simulink model "Simscape_Final_08042025"  (R2022a)
settings: Solver=VariableStepAuto  StartTime=0.0  StopTime=180  RelTol=1e-3  AbsTol=1e-3
libraries: fl_lib x30, sh_lib x20, nesl_utility x15, sdl_lib x3
settings Model: Creator=HP  LastModifiedBy=Abhishek
settings SolverCC: AutoScaleAbsTol=off  AlgebraicLoopSolver=TrustRegion  MaxZcPerStep=1
settings DebuggingCC: UnconnectedInputMsg=warning  UnconnectedOutputMsg=warning  UnconnectedLineMsg=warning  SymbolicDimsDataTypeCodeGenerationDiagnostic=none
settings SFSimCC: CustomCodeUndefinedFunction=UseInterfaceOnly
settings RTWCC: DLArmComputeVersion=19.05
settings SimscapeCC: SimscapeLogType=all  SimscapeLogSimulationStatistics=on  SimscapeLogDataHistory=10000

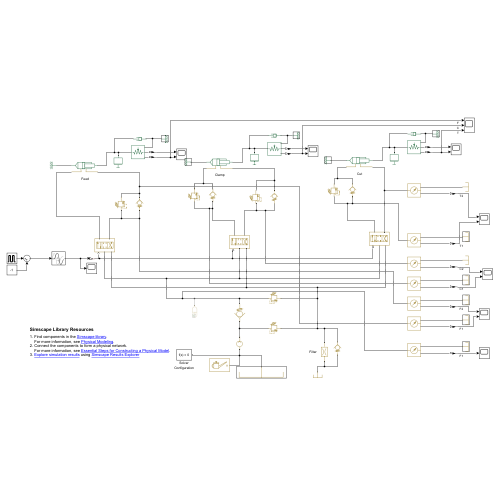
[thumbnail: Simulink's stored preview of the top-level diagram]
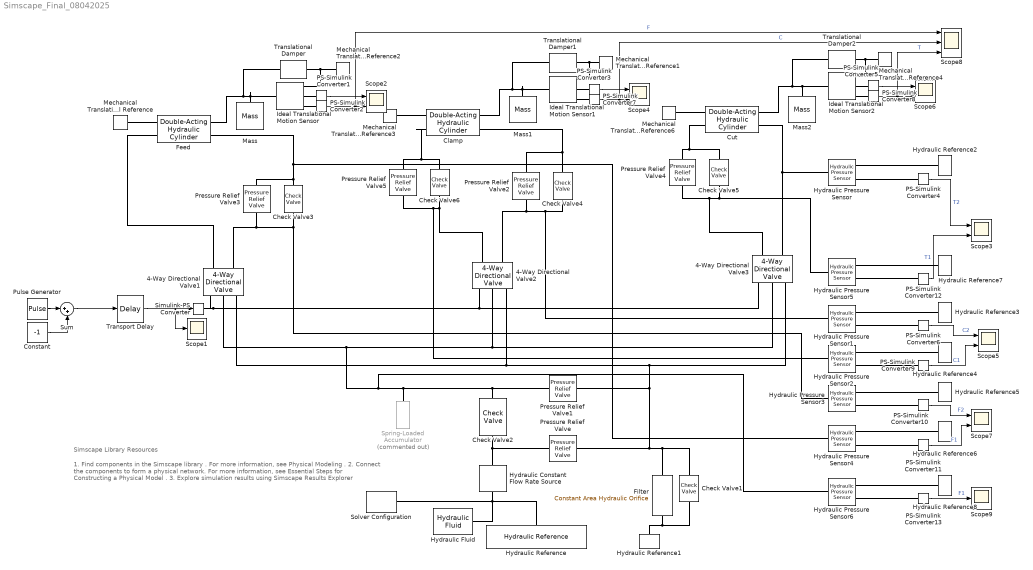
== system Simscape_Final_08042025 ==
  note: 1. Find components in the Simscape library .
      | For more information, see Physical Modeling .
      | 2. Connect the components to form a physical network.
      | For more information, see Essential Steps for Constructing a Physical Model .
      | 3. Explore simulation results using Simscape Results Explorer
  note: Simscape Library Resources
  4-Way Directional Valve1 : sh_lib/Valves/Directional Valves/4-Way Directional Valve  area_spec=sh.valves.directional_valves.enum.area_spec.identical  mdl_type_identical=sh.valves.directional_valves.enum.mdl_type.linear  mdl_type_different=sh.valves.directional_valves.enum.mdl_type.linear  interp_method_identical=sh.valves.directional_valves.enum.interp_method.linear  interp_method_different=sh.valves.directional_valves.enum.interp_method.linear  extrap_method_identical=sh.valves.directional_valves.enum.extrap_method.linear  extrap_method_different=sh.valves.directional_valves.enum.extrap_method.linear  A_leak=1e-12 m^2  C_d=0.7  lam_spec=sh.valves.directional_valves.enum.lam_spec.pressure_ratio  B_lam=0.999  Re_cr=12  opening_max=0.005 m  area_max=0.5e-4 m^2  opening_max_P_A=0.005 m  area_max_P_A=0.5e-4 m^2  opening_max_P_B=0.005 m  area_max_P_B=0.5e-4 m^2  opening_max_A_T=0.005 m  area_max_A_T=0.5e-4 m^2  opening_max_B_T=0.005 m  area_max_B_T=0.5e-4 m^2  opening_area_tab=[-.002, 0, .002, .005, .015] m  area_tab=[1e-09, 2.0352e-07, 4.0736e-05, .00011438, .00034356] m^2  opening_flow_rate_tab=[-.002, 0, .002, .005, .015] m  pressure_tab=[-10000000, -5000000, -2000000, 2000000, 5000000, 10000000] Pa  flow_rate_tab=[-1e-07, -7.0711e-08, -4.4721e-08, 4.4721e-08, 7.0711e-08, 1e-07; -2.0352e-05, -1.4391e-05, -9.1017e-06, 9.1017e-06, 1.4391e-05, 2.0352e-05; -.0040736, -.0028805, -.0018218, .0018218, .0028805, .0040736; -.011438, -.0080879, -.0051152, .0051152, .0080879, .011438; -.034356, -.024293, -.015364, .015364, .024293, .034356] m^3/s  opening_area_tab_P_A=[-.002, 0, .002, .005, .015] m  area_tab_P_A=[1e-09, 2.0352e-07, 4.0736e-05, .00011438, .00034356] m^2  opening_flow_rate_tab_P_A=[-.002, 0, .002, .005, .015] m  pressure_tab_P_A=[-10000000, -5000000, -2000000, 2000000, 5000000, 10000000] Pa  flow_rate_tab_P_A=[-1e-07, -7.0711e-08, -4.4721e-08, 4.4721e-08, 7.0711e-08, 1e-07; -2.0352e-05, -1.4391e-05, -9.1017e-06, 9.1017e-06, 1.4391e-05, 2.0352e-05; -.0040736, -.0028805, -.0018218, .0018218, .0028805, .0040736; -.011438, -.0080879, -.0051152, .0051152, .0080879, .011438; -.034356, -.024293, -.015364, .015364, .024293, .034356] m^3/s  opening_area_tab_P_B=[-.002, 0, .002, .005, .015] m  area_tab_P_B=[1e-09, 2.0352e-07, 4.0736e-05, .00011438, .00034356] m^2  opening_flow_rate_tab_P_B=[-.002, 0, .002, .005, .015] m  pressure_tab_P_B=[-10000000, -5000000, -2000000, 2000000, 5000000, 10000000] Pa  flow_rate_tab_P_B=[-1e-07, -7.0711e-08, -4.4721e-08, 4.4721e-08, 7.0711e-08, 1e-07; -2.0352e-05, -1.4391e-05, -9.1017e-06, 9.1017e-06, 1.4391e-05, 2.0352e-05; -.0040736, -.0028805, -.0018218, .0018218, .0028805, .0040736; -.011438, -.0080879, -.0051152, .0051152, .0080879, .011438; -.034356, -.024293, -.015364, .015364, .024293, .034356] m^3/s  opening_area_tab_A_T=[-.002, 0, .002, .005, .015] m  area_tab_A_T=[1e-09, 2.0352e-07, 4.0736e-05, .00011438, .00034356] m^2  opening_flow_rate_tab_A_T=[-.002, 0, .002, .005, .015] m  pressure_tab_A_T=[-10000000, -5000000, -2000000, 2000000, 5000000, 10000000] Pa  flow_rate_tab_A_T=[-1e-07, -7.0711e-08, -4.4721e-08, 4.4721e-08, 7.0711e-08, 1e-07; -2.0352e-05, -1.4391e-05, -9.1017e-06, 9.1017e-06, 1.4391e-05, 2.0352e-05; -.0040736, -.0028805, -.0018218, .0018218, .0028805, .0040736; -.011438, -.0080879, -.0051152, .0051152, .0080879, .011438; -.034356, -.024293, -.015364, .015364, .024293, .034356] m^3/s  opening_area_tab_B_T=[-.002, 0, .002, .005, .015] m  area_tab_B_T=[1e-09, 2.0352e-07, 4.0736e-05, .00011438, .00034356] m^2  opening_flow_rate_tab_B_T=[-.002, 0, .002, .005, .015] m  pressure_tab_B_T=[-10000000, -5000000, -2000000, 2000000, 5000000, 10000000] Pa  flow_rate_tab_B_T=[-1e-07, -7.0711e-08, -4.4721e-08, 4.4721e-08, 7.0711e-08, 1e-07; -2.0352e-05, -1.4391e-05, -9.1017e-06, 9.1017e-06, 1.4391e-05, 2.0352e-05; -.0040736, -.0028805, -.0018218, .0018218, .0028805, .0040736; -.011438, -.0080879, -.0051152, .0051152, .0080879, .011438; -.034356, -.024293, -.015364, .015364, .024293, .034356] m^3/s  x_0_P_A=0 m  x_0_P_B=0 m  x_0_A_T=0 m  x_0_B_T=0 m
      settings: LogSimulationData=on  InternalSimscapePortConfiguration="{\"Bottom\":[],\"Left\":[{\"id\":\"A\",\"label\":\"A\",\"type\":\"foundation.hydraulic.hydraulic\"},{\"id\":\"B\",\"label\":\"B\",\"type\":\"foundation.hydraulic.hydraulic\"}],\"Right\":[{\"id\":\"S\",\"label\":\"S\",\"type\":\"input\"},{\"id\":\"P\",\"label\":\"P\",\"type\":\"foundation.hydraulic.hydraulic\"},{\"id\":\"T\",\"label\":\"T\",\"type\":\"foundation.hydraulic.hydraulic\"}],\"Top\":[]}"
  4-Way Directional Valve2 : sh_lib/Valves/Directional Valves/4-Way Directional Valve  area_spec=sh.valves.directional_valves.enum.area_spec.identical  mdl_type_identical=sh.valves.directional_valves.enum.mdl_type.linear  mdl_type_different=sh.valves.directional_valves.enum.mdl_type.linear  interp_method_identical=sh.valves.directional_valves.enum.interp_method.linear  interp_method_different=sh.valves.directional_valves.enum.interp_method.linear  extrap_method_identical=sh.valves.directional_valves.enum.extrap_method.linear  extrap_method_different=sh.valves.directional_valves.enum.extrap_method.linear  A_leak=1e-12 m^2  C_d=0.7  lam_spec=sh.valves.directional_valves.enum.lam_spec.pressure_ratio  B_lam=0.999  Re_cr=12  opening_max=0.005 m  area_max=0.5e-4 m^2  opening_max_P_A=0.005 m  area_max_P_A=0.5e-4 m^2  opening_max_P_B=0.005 m  area_max_P_B=0.5e-4 m^2  opening_max_A_T=0.005 m  area_max_A_T=0.5e-4 m^2  opening_max_B_T=0.005 m  area_max_B_T=0.5e-4 m^2  opening_area_tab=[-.002, 0, .002, .005, .015] m  area_tab=[1e-09, 2.0352e-07, 4.0736e-05, .00011438, .00034356] m^2  opening_flow_rate_tab=[-.002, 0, .002, .005, .015] m  pressure_tab=[-10000000, -5000000, -2000000, 2000000, 5000000, 10000000] Pa  flow_rate_tab=[-1e-07, -7.0711e-08, -4.4721e-08, 4.4721e-08, 7.0711e-08, 1e-07; -2.0352e-05, -1.4391e-05, -9.1017e-06, 9.1017e-06, 1.4391e-05, 2.0352e-05; -.0040736, -.0028805, -.0018218, .0018218, .0028805, .0040736; -.011438, -.0080879, -.0051152, .0051152, .0080879, .011438; -.034356, -.024293, -.015364, .015364, .024293, .034356] m^3/s  opening_area_tab_P_A=[-.002, 0, .002, .005, .015] m  area_tab_P_A=[1e-09, 2.0352e-07, 4.0736e-05, .00011438, .00034356] m^2  opening_flow_rate_tab_P_A=[-.002, 0, .002, .005, .015] m  pressure_tab_P_A=[-10000000, -5000000, -2000000, 2000000, 5000000, 10000000] Pa  flow_rate_tab_P_A=[-1e-07, -7.0711e-08, -4.4721e-08, 4.4721e-08, 7.0711e-08, 1e-07; -2.0352e-05, -1.4391e-05, -9.1017e-06, 9.1017e-06, 1.4391e-05, 2.0352e-05; -.0040736, -.0028805, -.0018218, .0018218, .0028805, .0040736; -.011438, -.0080879, -.0051152, .0051152, .0080879, .011438; -.034356, -.024293, -.015364, .015364, .024293, .034356] m^3/s  opening_area_tab_P_B=[-.002, 0, .002, .005, .015] m  area_tab_P_B=[1e-09, 2.0352e-07, 4.0736e-05, .00011438, .00034356] m^2  opening_flow_rate_tab_P_B=[-.002, 0, .002, .005, .015] m  pressure_tab_P_B=[-10000000, -5000000, -2000000, 2000000, 5000000, 10000000] Pa  flow_rate_tab_P_B=[-1e-07, -7.0711e-08, -4.4721e-08, 4.4721e-08, 7.0711e-08, 1e-07; -2.0352e-05, -1.4391e-05, -9.1017e-06, 9.1017e-06, 1.4391e-05, 2.0352e-05; -.0040736, -.0028805, -.0018218, .0018218, .0028805, .0040736; -.011438, -.0080879, -.0051152, .0051152, .0080879, .011438; -.034356, -.024293, -.015364, .015364, .024293, .034356] m^3/s  opening_area_tab_A_T=[-.002, 0, .002, .005, .015] m  area_tab_A_T=[1e-09, 2.0352e-07, 4.0736e-05, .00011438, .00034356] m^2  opening_flow_rate_tab_A_T=[-.002, 0, .002, .005, .015] m  pressure_tab_A_T=[-10000000, -5000000, -2000000, 2000000, 5000000, 10000000] Pa  flow_rate_tab_A_T=[-1e-07, -7.0711e-08, -4.4721e-08, 4.4721e-08, 7.0711e-08, 1e-07; -2.0352e-05, -1.4391e-05, -9.1017e-06, 9.1017e-06, 1.4391e-05, 2.0352e-05; -.0040736, -.0028805, -.0018218, .0018218, .0028805, .0040736; -.011438, -.0080879, -.0051152, .0051152, .0080879, .011438; -.034356, -.024293, -.015364, .015364, .024293, .034356] m^3/s  opening_area_tab_B_T=[-.002, 0, .002, .005, .015] m  area_tab_B_T=[1e-09, 2.0352e-07, 4.0736e-05, .00011438, .00034356] m^2  opening_flow_rate_tab_B_T=[-.002, 0, .002, .005, .015] m  pressure_tab_B_T=[-10000000, -5000000, -2000000, 2000000, 5000000, 10000000] Pa  flow_rate_tab_B_T=[-1e-07, -7.0711e-08, -4.4721e-08, 4.4721e-08, 7.0711e-08, 1e-07; -2.0352e-05, -1.4391e-05, -9.1017e-06, 9.1017e-06, 1.4391e-05, 2.0352e-05; -.0040736, -.0028805, -.0018218, .0018218, .0028805, .0040736; -.011438, -.0080879, -.0051152, .0051152, .0080879, .011438; -.034356, -.024293, -.015364, .015364, .024293, .034356] m^3/s  x_0_P_A=0 m  x_0_P_B=0 m  x_0_A_T=0 m  x_0_B_T=0 m
      settings: LogSimulationData=on  InternalSimscapePortConfiguration="{\"Bottom\":[],\"Left\":[{\"id\":\"A\",\"label\":\"A\",\"type\":\"foundation.hydraulic.hydraulic\"},{\"id\":\"B\",\"label\":\"B\",\"type\":\"foundation.hydraulic.hydraulic\"}],\"Right\":[{\"id\":\"S\",\"label\":\"S\",\"type\":\"input\"},{\"id\":\"P\",\"label\":\"P\",\"type\":\"foundation.hydraulic.hydraulic\"},{\"id\":\"T\",\"label\":\"T\",\"type\":\"foundation.hydraulic.hydraulic\"}],\"Top\":[]}"
  4-Way Directional Valve3 : sh_lib/Valves/Directional Valves/4-Way Directional Valve  area_spec=sh.valves.directional_valves.enum.area_spec.identical  mdl_type_identical=sh.valves.directional_valves.enum.mdl_type.linear  mdl_type_different=sh.valves.directional_valves.enum.mdl_type.linear  interp_method_identical=sh.valves.directional_valves.enum.interp_method.linear  interp_method_different=sh.valves.directional_valves.enum.interp_method.linear  extrap_method_identical=sh.valves.directional_valves.enum.extrap_method.linear  extrap_method_different=sh.valves.directional_valves.enum.extrap_method.linear  A_leak=1e-12 m^2  C_d=0.7  lam_spec=sh.valves.directional_valves.enum.lam_spec.pressure_ratio  B_lam=0.999  Re_cr=12  opening_max=0.005 m  area_max=0.5e-4 m^2  opening_max_P_A=0.005 m  area_max_P_A=0.5e-4 m^2  opening_max_P_B=0.005 m  area_max_P_B=0.5e-4 m^2  opening_max_A_T=0.005 m  area_max_A_T=0.5e-4 m^2  opening_max_B_T=0.005 m  area_max_B_T=0.5e-4 m^2  opening_area_tab=[-.002, 0, .002, .005, .015] m  area_tab=[1e-09, 2.0352e-07, 4.0736e-05, .00011438, .00034356] m^2  opening_flow_rate_tab=[-.002, 0, .002, .005, .015] m  pressure_tab=[-10000000, -5000000, -2000000, 2000000, 5000000, 10000000] Pa  flow_rate_tab=[-1e-07, -7.0711e-08, -4.4721e-08, 4.4721e-08, 7.0711e-08, 1e-07; -2.0352e-05, -1.4391e-05, -9.1017e-06, 9.1017e-06, 1.4391e-05, 2.0352e-05; -.0040736, -.0028805, -.0018218, .0018218, .0028805, .0040736; -.011438, -.0080879, -.0051152, .0051152, .0080879, .011438; -.034356, -.024293, -.015364, .015364, .024293, .034356] m^3/s  opening_area_tab_P_A=[-.002, 0, .002, .005, .015] m  area_tab_P_A=[1e-09, 2.0352e-07, 4.0736e-05, .00011438, .00034356] m^2  opening_flow_rate_tab_P_A=[-.002, 0, .002, .005, .015] m  pressure_tab_P_A=[-10000000, -5000000, -2000000, 2000000, 5000000, 10000000] Pa  flow_rate_tab_P_A=[-1e-07, -7.0711e-08, -4.4721e-08, 4.4721e-08, 7.0711e-08, 1e-07; -2.0352e-05, -1.4391e-05, -9.1017e-06, 9.1017e-06, 1.4391e-05, 2.0352e-05; -.0040736, -.0028805, -.0018218, .0018218, .0028805, .0040736; -.011438, -.0080879, -.0051152, .0051152, .0080879, .011438; -.034356, -.024293, -.015364, .015364, .024293, .034356] m^3/s  opening_area_tab_P_B=[-.002, 0, .002, .005, .015] m  area_tab_P_B=[1e-09, 2.0352e-07, 4.0736e-05, .00011438, .00034356] m^2  opening_flow_rate_tab_P_B=[-.002, 0, .002, .005, .015] m  pressure_tab_P_B=[-10000000, -5000000, -2000000, 2000000, 5000000, 10000000] Pa  flow_rate_tab_P_B=[-1e-07, -7.0711e-08, -4.4721e-08, 4.4721e-08, 7.0711e-08, 1e-07; -2.0352e-05, -1.4391e-05, -9.1017e-06, 9.1017e-06, 1.4391e-05, 2.0352e-05; -.0040736, -.0028805, -.0018218, .0018218, .0028805, .0040736; -.011438, -.0080879, -.0051152, .0051152, .0080879, .011438; -.034356, -.024293, -.015364, .015364, .024293, .034356] m^3/s  opening_area_tab_A_T=[-.002, 0, .002, .005, .015] m  area_tab_A_T=[1e-09, 2.0352e-07, 4.0736e-05, .00011438, .00034356] m^2  opening_flow_rate_tab_A_T=[-.002, 0, .002, .005, .015] m  pressure_tab_A_T=[-10000000, -5000000, -2000000, 2000000, 5000000, 10000000] Pa  flow_rate_tab_A_T=[-1e-07, -7.0711e-08, -4.4721e-08, 4.4721e-08, 7.0711e-08, 1e-07; -2.0352e-05, -1.4391e-05, -9.1017e-06, 9.1017e-06, 1.4391e-05, 2.0352e-05; -.0040736, -.0028805, -.0018218, .0018218, .0028805, .0040736; -.011438, -.0080879, -.0051152, .0051152, .0080879, .011438; -.034356, -.024293, -.015364, .015364, .024293, .034356] m^3/s  opening_area_tab_B_T=[-.002, 0, .002, .005, .015] m  area_tab_B_T=[1e-09, 2.0352e-07, 4.0736e-05, .00011438, .00034356] m^2  opening_flow_rate_tab_B_T=[-.002, 0, .002, .005, .015] m  pressure_tab_B_T=[-10000000, -5000000, -2000000, 2000000, 5000000, 10000000] Pa  flow_rate_tab_B_T=[-1e-07, -7.0711e-08, -4.4721e-08, 4.4721e-08, 7.0711e-08, 1e-07; -2.0352e-05, -1.4391e-05, -9.1017e-06, 9.1017e-06, 1.4391e-05, 2.0352e-05; -.0040736, -.0028805, -.0018218, .0018218, .0028805, .0040736; -.011438, -.0080879, -.0051152, .0051152, .0080879, .011438; -.034356, -.024293, -.015364, .015364, .024293, .034356] m^3/s  x_0_P_A=0 m  x_0_P_B=0 m  x_0_A_T=0 m  x_0_B_T=0 m
      settings: LogSimulationData=on  InternalSimscapePortConfiguration="{\"Bottom\":[],\"Left\":[{\"id\":\"A\",\"label\":\"A\",\"type\":\"foundation.hydraulic.hydraulic\"},{\"id\":\"B\",\"label\":\"B\",\"type\":\"foundation.hydraulic.hydraulic\"}],\"Right\":[{\"id\":\"S\",\"label\":\"S\",\"type\":\"input\"},{\"id\":\"P\",\"label\":\"P\",\"type\":\"foundation.hydraulic.hydraulic\"},{\"id\":\"T\",\"label\":\"T\",\"type\":\"foundation.hydraulic.hydraulic\"}],\"Top\":[]}"
  Check Valve{1..6} (6 alike) : sh_lib/Valves/Directional Valves/Check Valve  area_max=1e-4 m^2  pres_crack=0.3e5 Pa  pres_max=1.2e5 Pa  C_d=0.7  A_leak=1e-12 m^2  lam_spec=1  B_lam=0.999  Re_cr=12  dynamic=0  tau=0.1 s  area_init=1e-12 m^2
      settings: InternalSimscapePortConfiguration="{\"Bottom\":[],\"Left\":[{\"id\":\"A\",\"label\":\"A\",\"type\":\"foundation.hydraulic.hydraulic\"}],\"Right\":[{\"id\":\"B\",\"label\":\"B\",\"type\":\"foundation.hydraulic.hydraulic\"}],\"Top\":[]}"
  Clamp : sh_lib/Hydraulic Cylinders/Double-Acting Hydraulic Cylinder  area_A=1256.6 mm^2  area_B=876.9 mm^2  stroke=150 mm  dead_vol_A=1e-4 m^3  dead_vol_B=1e-4 m^3  k_sh=1.4  or=sh.cylinders.enum.MechOrientationTranslational.Positive  stiff=1e6 N/m  D=150 N*s/m  hardstop_model=1  transition=0.1 mm  displacement_spec=foundation.enum.DisplacementSpec.Calculate  init_pos=0 m  init_pressure_A=0 Pa  init_pressure_B=0 Pa
      settings: InternalSimscapePortConfiguration="{\"Bottom\":[],\"Left\":[{\"id\":\"C\",\"label\":\"C\",\"type\":\"foundation.mechanical.translational.translational\"},{\"id\":\"A\",\"label\":\"A\",\"type\":\"foundation.hydraulic.hydraulic\"}],\"Right\":[{\"id\":\"R\",\"label\":\"R\",\"type\":\"foundation.mechanical.translational.translational\"},{\"id\":\"B\",\"label\":\"B\",\"type\":\"foundation.hydraulic.hydraulic\"}],\"Top\":[]}"
  Constant : Constant  Value=-1
  Cut : sh_lib/Hydraulic Cylinders/Double-Acting Hydraulic Cylinder  area_A=1256.6 mm^2  area_B=876.9 mm^2  stroke=250 mm  dead_vol_A=1e-4 m^3  dead_vol_B=1e-4 m^3  k_sh=1.4  or=sh.cylinders.enum.MechOrientationTranslational.Positive  stiff=1e6 N/m  D=150 N*s/m  hardstop_model=1  transition=0.1 mm  displacement_spec=foundation.enum.DisplacementSpec.Calculate  init_pos=0 m  init_pressure_A=0 Pa  init_pressure_B=0 Pa
      settings: InternalSimscapePortConfiguration="{\"Bottom\":[],\"Left\":[{\"id\":\"C\",\"label\":\"C\",\"type\":\"foundation.mechanical.translational.translational\"},{\"id\":\"A\",\"label\":\"A\",\"type\":\"foundation.hydraulic.hydraulic\"}],\"Right\":[{\"id\":\"R\",\"label\":\"R\",\"type\":\"foundation.mechanical.translational.translational\"},{\"id\":\"B\",\"label\":\"B\",\"type\":\"foundation.hydraulic.hydraulic\"}],\"Top\":[]}"
  Feed : sh_lib/Hydraulic Cylinders/Double-Acting Hydraulic Cylinder  area_A=1256.6 mm^2  area_B=876.9 mm^2  stroke=200 mm  dead_vol_A=1e-4 m^3  dead_vol_B=1e-4 m^3  k_sh=1.4  or=sh.cylinders.enum.MechOrientationTranslational.Positive  stiff=1e6 N/m  D=150 N*s/m  hardstop_model=1  transition=0.1 mm  displacement_spec=foundation.enum.DisplacementSpec.Calculate  init_pos=0 m  init_pressure_A=0 Pa  init_pressure_B=0 Pa
      settings: InternalSimscapePortConfiguration="{\"Bottom\":[],\"Left\":[{\"id\":\"C\",\"label\":\"C\",\"type\":\"foundation.mechanical.translational.translational\"},{\"id\":\"A\",\"label\":\"A\",\"type\":\"foundation.hydraulic.hydraulic\"}],\"Right\":[{\"id\":\"R\",\"label\":\"R\",\"type\":\"foundation.mechanical.translational.translational\"},{\"id\":\"B\",\"label\":\"B\",\"type\":\"foundation.hydraulic.hydraulic\"}],\"Top\":[]}"
  "Filter " : fl_lib/Hydraulic/Hydraulic Elements/Constant Area Hydraulic Orifice  area=1e-4 m^2  C_d=0.7  lam_spec=1  B_lam=0.999  Re_cr=12  q_specify=off  q_priority=None  q=1e-3 m^3/s  q_nominal_specify=off  q_nominal_unit=m^3/s  q_nominal_value=1  p_specify=off  p_priority=None  p=0 Pa  p_nominal_specify=off  p_nominal_unit=Pa  p_nominal_value=1
      settings: InternalSimscapePortConfiguration="{\"Bottom\":[],\"Left\":[{\"id\":\"A\",\"label\":\"A\",\"type\":\"foundation.hydraulic.hydraulic\"}],\"Right\":[{\"id\":\"B\",\"label\":\"B\",\"type\":\"foundation.hydraulic.hydraulic\"}],\"Top\":[]}"
  Hydraulic Constant Flow Rate Source : fl_lib/Hydraulic/Hydraulic Sources/Hydraulic Constant Flow Rate Source  commanded_flow_rate=1.666*0.1*3 gpm
      settings: InternalSimscapePortConfiguration="{\"Bottom\":[],\"Left\":[{\"id\":\"P\",\"label\":\"P\",\"type\":\"foundation.hydraulic.hydraulic\"}],\"Right\":[{\"id\":\"T\",\"label\":\"T\",\"type\":\"foundation.hydraulic.hydraulic\"}],\"Top\":[]}"
  Hydraulic Fluid : sh_lib/Hydraulic Utilities/Hydraulic Fluid  SelFluid=1  SysTemp=60  TrapAir=0.005  ViscDerFactor=1  range_error=2
  Hydraulic Pressure Sensor{,1..6} (7 alike) : fl_lib/Hydraulic/Hydraulic Sensors/Hydraulic Pressure Sensor
  Hydraulic Reference{,1..8} (9 alike) : fl_lib/Hydraulic/Hydraulic Elements/Hydraulic Reference
  Ideal Translational Motion Sensor : fl_lib/Mechanical/Mechanical Sensors/Ideal Translational Motion Sensor  reference=foundation.enum.MeasurementReference.difference  acceleration_port=false  velocity_port=true  position_port=true  offset=0 m
  Ideal Translational Motion Sensor1 : fl_lib/Mechanical/Mechanical Sensors/Ideal Translational Motion Sensor  reference=foundation.enum.MeasurementReference.difference  acceleration_port=false  velocity_port=true  position_port=true  offset=0 m
  Ideal Translational Motion Sensor2 : fl_lib/Mechanical/Mechanical Sensors/Ideal Translational Motion Sensor  reference=foundation.enum.MeasurementReference.difference  acceleration_port=false  velocity_port=true  position_port=true  offset=0 m
  Mass : fl_lib/Mechanical/Translational Elements/Mass  mass=10 kg  num_ports=foundation.enum.numPorts2.one  v_specify=off  v_priority=High  v=0 m/s  v_nominal_specify=off  v_nominal_unit=m/s  v_nominal_value=1  f_specify=off  f_priority=None  f=0 N  f_nominal_specify=off  f_nominal_unit=N  f_nominal_value=1
  Mass1 : fl_lib/Mechanical/Translational Elements/Mass  mass=40 kg  num_ports=foundation.enum.numPorts2.one  v_specify=off  v_priority=High  v=0 m/s  v_nominal_specify=off  v_nominal_unit=m/s  v_nominal_value=1  f_specify=off  f_priority=None  f=0 N  f_nominal_specify=off  f_nominal_unit=N  f_nominal_value=1
  Mass2 : fl_lib/Mechanical/Translational Elements/Mass  mass=80 kg  num_ports=foundation.enum.numPorts2.one  v_specify=off  v_priority=High  v=0 m/s  v_nominal_specify=off  v_nominal_unit=m/s  v_nominal_value=1  f_specify=off  f_priority=None  f=0 N  f_nominal_specify=off  f_nominal_unit=N  f_nominal_value=1
  Mechanical Translational Reference{,1..4,6} (6 alike) : fl_lib/Mechanical/Translational Elements/Mechanical Translational Reference
  PS-Simulink Converter{1..13} (13 alike) : nesl_utility/PS-Simulink Converter  PhysicalDomain=network_engine_domain  SubClassName=ps_output  LeftPortType=input  RightPortType=output  PseudoPeriodic=off  Frequencies=[]  VectorFormat=inherit  Unit=inherit  AffineConversion=off
  Pressure Relief Valve : sh_lib/Valves/Pressure Control Valves/Pressure Relief Valve  valve_area_spec=1  p_diff_TLU=[30.15e5 : 15e3 : 31.35e5] Pa  area_TLU=[1 : 1 : 9] .* 1e-5 m^2  area_max=1e-4 m^2  pres_set=1000 kPa  reg_range=1000*0.2 kPa  C_d=0.7  A_leak=1e-12 m^2  lam_spec=1  B_lam=0.999  Re_cr=12  dynamic=0  tau=0.1 s  area_init=1e-12 m^2
      settings: InternalSimscapePortConfiguration="{\"Bottom\":[],\"Left\":[{\"id\":\"A\",\"label\":\"A\",\"type\":\"foundation.hydraulic.hydraulic\"}],\"Right\":[{\"id\":\"B\",\"label\":\"B\",\"type\":\"foundation.hydraulic.hydraulic\"}],\"Top\":[]}"
  Pressure Relief Valve1 : sh_lib/Valves/Pressure Control Valves/Pressure Relief Valve  valve_area_spec=1  p_diff_TLU=[30.15e5 : 15e3 : 31.35e5] Pa  area_TLU=[1 : 1 : 9] .* 1e-5 m^2  area_max=1e-4 m^2  pres_set=900 kPa  reg_range=900*0.2 kPa  C_d=0.7  A_leak=1e-12 m^2  lam_spec=1  B_lam=0.999  Re_cr=12  dynamic=0  tau=0.1 s  area_init=1e-12 m^2
      settings: InternalSimscapePortConfiguration="{\"Bottom\":[],\"Left\":[{\"id\":\"A\",\"label\":\"A\",\"type\":\"foundation.hydraulic.hydraulic\"}],\"Right\":[{\"id\":\"B\",\"label\":\"B\",\"type\":\"foundation.hydraulic.hydraulic\"}],\"Top\":[]}"
  Pressure Relief Valve2 : sh_lib/Valves/Pressure Control Valves/Pressure Relief Valve  valve_area_spec=1  p_diff_TLU=[30.15e5 : 15e3 : 31.35e5] Pa  area_TLU=[1 : 1 : 9] .* 1e-5 m^2  area_max=1e-4 m^2  pres_set=456 kPa  reg_range=456*0.2 kPa  C_d=0.7  A_leak=1e-12 m^2  lam_spec=1  B_lam=0.999  Re_cr=12  dynamic=0  tau=0.1 s  area_init=1e-12 m^2
      settings: InternalSimscapePortConfiguration="{\"Bottom\":[],\"Left\":[{\"id\":\"A\",\"label\":\"A\",\"type\":\"foundation.hydraulic.hydraulic\"}],\"Right\":[{\"id\":\"B\",\"label\":\"B\",\"type\":\"foundation.hydraulic.hydraulic\"}],\"Top\":[]}"
  Pressure Relief Valve3 : sh_lib/Valves/Pressure Control Valves/Pressure Relief Valve  valve_area_spec=1  p_diff_TLU=[30.15e5 : 15e3 : 31.35e5] Pa  area_TLU=[1 : 1 : 9] .* 1e-5 m^2  area_max=1e-4 m^2  pres_set=750 kPa  reg_range=750*0.2 kPa  C_d=0.7  A_leak=1e-12 m^2  lam_spec=1  B_lam=0.999  Re_cr=12  dynamic=0  tau=0.1 s  area_init=1e-12 m^2
      settings: InternalSimscapePortConfiguration="{\"Bottom\":[],\"Left\":[{\"id\":\"A\",\"label\":\"A\",\"type\":\"foundation.hydraulic.hydraulic\"}],\"Right\":[{\"id\":\"B\",\"label\":\"B\",\"type\":\"foundation.hydraulic.hydraulic\"}],\"Top\":[]}"
  Pressure Relief Valve4 : sh_lib/Valves/Pressure Control Valves/Pressure Relief Valve  valve_area_spec=1  p_diff_TLU=[30.15e5 : 15e3 : 31.35e5] Pa  area_TLU=[1 : 1 : 9] .* 1e-5 m^2  area_max=1e-4 m^2  pres_set=637 kPa  reg_range=127.4 kPa  C_d=0.7  A_leak=1e-12 m^2  lam_spec=1  B_lam=0.999  Re_cr=12  dynamic=0  tau=0.1 s  area_init=1e-12 m^2
      settings: InternalSimscapePortConfiguration="{\"Bottom\":[],\"Left\":[{\"id\":\"A\",\"label\":\"A\",\"type\":\"foundation.hydraulic.hydraulic\"}],\"Right\":[{\"id\":\"B\",\"label\":\"B\",\"type\":\"foundation.hydraulic.hydraulic\"}],\"Top\":[]}"
  Pressure Relief Valve5 : sh_lib/Valves/Pressure Control Valves/Pressure Relief Valve  valve_area_spec=1  p_diff_TLU=[30.15e5 : 15e3 : 31.35e5] Pa  area_TLU=[1 : 1 : 9] .* 1e-5 m^2  area_max=1e-4 m^2  pres_set=318 kPa  reg_range=63 kPa  C_d=0.7  A_leak=1e-12 m^2  lam_spec=1  B_lam=0.999  Re_cr=12  dynamic=0  tau=0.1 s  area_init=1e-12 m^2
      settings: InternalSimscapePortConfiguration="{\"Bottom\":[],\"Left\":[{\"id\":\"A\",\"label\":\"A\",\"type\":\"foundation.hydraulic.hydraulic\"}],\"Right\":[{\"id\":\"B\",\"label\":\"B\",\"type\":\"foundation.hydraulic.hydraulic\"}],\"Top\":[]}"
  Pulse Generator : DiscretePulseGenerator  PulseType=Time based  Amplitude=2  Period=60  PulseWidth=50  PhaseDelay=1
  Scope1 : Scope
  Scope{2..7} (6 alike) : Scope  NumInputPorts=2
  Scope8 : Scope  NumInputPorts=3
  Scope9 : Scope
  Simulink-PS Converter : nesl_utility/Simulink-PS Converter  PhysicalDomain=network_engine_domain  SubClassName=ps_input  LeftPortType=input  RightPortType=output  PseudoPeriodic=off  Frequencies=[]  NoiseDistribution=none  NoiseParameters=[]  Unit=1  AffineConversion=off  FilteringAndDerivatives=provide  SimscapeFilterOrder=1  InputFilterTimeConstant=0.001  UdotUserProvided=0
  Solver Configuration : nesl_utility/Solver Configuration  PhysicalDomain=network_engine_domain  SubClassName=solver  LeftPortType=input  RightPortType=generic  Tones=[]  Harmonics=[]  SimulateNoise=off  Profile=off  UseLocalSampling=off  EnableSwitchedLinearOptims=on  FrequencyDomain=off  UseCCode=off  RelTol=0.001  AbsTol=1e-06  MinStep=1e-09  ToWorkspace=off  RevertToSquareIcSolve=off  NumHomotopyIterations=100  PhasorMode=off  PhasorModeNumHarmonics=1  ConsistencySolver=NEWTON_XTOL_AFTER_FTOL  IndexReductionMethod=DerivativeReplacement  DoDC=off  ResidualTolerance=1e-09  ConsistencyTolSource=GLOBAL  ConsistencyAbsTol=0.001  ConsistencyRelTol=0.001  ConsistencyTolFactor=0.001  UseLocalSolver=off  LocalSolverChoice=NE_BACKWARD_EULER_ADVANCER  ResolveIndetEquations=on  FunctionEvalNumThread=1  LocalSolverSampleTime=0.001  DoFixedCost=off  MaxNonlinIter=3  MaxModeIter=2  ComputeImpulses=off  ImpulseIterations=2  LinearAlgebra=auto  LinearAlgebraNumThread=0  EquationFormulation=NE_TIME_EF  DelaysMemoryBudget=1024  AutomaticFiltering=on  FilteringTimeConstant=0.001  PartitionStorageMethod=AS_NEEDED  PartitionMemoryBudget=1024  PartitionMethod=ROBUST  MultibodyUseLocalSolver=off  MultibodyLocalSolverChoice=ODE1  MultibodyLocalSolverSampleTime=0.001
  Spring-Loaded Accumulator : sh_lib/Accumulators/Spring-Loaded Accumulator  Commented=on  capacity=8 l  pr_preload=400 kPa  pr_max=760 kPa  stiff_coeff=1e12 Pa/m^3  penetr_coeff=1e10 Pa*s/m^6  flow_rate_specify=off  flow_rate_priority=None  flow_rate=5e-3 m^3/s  flow_rate_nominal_specify=off  flow_rate_nominal_unit=m^3/s  flow_rate_nominal_value=1  fluid_volume_specify=on  fluid_volume_priority=High  fluid_volume=5e-3 m^3  fluid_volume_nominal_specify=off  fluid_volume_nominal_unit=m^3  fluid_volume_nominal_value=1  fluid_pressure_specify=off  fluid_pressure_priority=None  fluid_pressure=1.01325e5 Pa  fluid_pressure_nominal_specify=off  fluid_pressure_nominal_unit=Pa  fluid_pressure_nominal_value=1
      settings: InternalSimscapePortConfiguration="{\"Bottom\":[],\"Left\":[],\"Right\":[{\"id\":\"A\",\"label\":\"A\",\"type\":\"foundation.hydraulic.hydraulic\"}],\"Top\":[]}"
  Sum : Sum  Inputs=|++
  Translational Damper : sdl_lib/Couplings & Drives/Springs & Dampers/Translational Damper  D=1000 N*s/m  enable_faults=simscape.enum.onoff.off  b_fault=1e6 N*s/m  temporal_fault=simscape.enum.onoff.off  fault_time=5 s  shock_fault=simscape.enum.onoff.off  acceleration_limit=100 m/s^2  shock_limit=1  report_fault=simscape.enum.assert.action.none  thermal_port=simscape.enum.thermaleffects.omit  thermal_mass=50 kJ/K  temperature_specify=off  temperature_priority=High  temperature=300 K  temperature_nominal_specify=off  temperature_nominal_unit=K  temperature_nominal_value=1
  Translational Damper1 : sdl_lib/Couplings & Drives/Springs & Dampers/Translational Damper  D=1000 N*s/m  enable_faults=simscape.enum.onoff.off  b_fault=1e6 N*s/m  temporal_fault=simscape.enum.onoff.off  fault_time=5 s  shock_fault=simscape.enum.onoff.off  acceleration_limit=100 m/s^2  shock_limit=1  report_fault=simscape.enum.assert.action.none  thermal_port=simscape.enum.thermaleffects.omit  thermal_mass=50 kJ/K  temperature_specify=off  temperature_priority=High  temperature=300 K  temperature_nominal_specify=off  temperature_nominal_unit=K  temperature_nominal_value=1
  Translational Damper2 : sdl_lib/Couplings & Drives/Springs & Dampers/Translational Damper  D=1100 N*s/m  enable_faults=simscape.enum.onoff.off  b_fault=1e6 N*s/m  temporal_fault=simscape.enum.onoff.off  fault_time=5 s  shock_fault=simscape.enum.onoff.off  acceleration_limit=100 m/s^2  shock_limit=1  report_fault=simscape.enum.assert.action.none  thermal_port=simscape.enum.thermaleffects.omit  thermal_mass=50 kJ/K  temperature_specify=off  temperature_priority=High  temperature=300 K  temperature_nominal_specify=off  temperature_nominal_unit=K  temperature_nominal_value=1
  Transport Delay : TransportDelay  DelayTime=60
  wires:
  Constant/1 -> Sum/2
  Sum/1 -> Transport Delay/1
  Pulse Generator/1 -> Sum/1
  PS-Simulink Converter1/1 -> Scope2/1
  PS-Simulink Converter7/1 -> Scope8/2, Scope4/2  "C"
  PS-Simulink Converter3/1 -> Scope4/1
  PS-Simulink Converter8/1 -> Scope8/3, Scope6/2  "T"
  PS-Simulink Converter5/1 -> Scope6/1
  PS-Simulink Converter2/1 -> Scope8/1, Scope2/2  "F"
  PS-Simulink Converter4/1 -> Scope3/1  "T2"
  PS-Simulink Converter6/1 -> Scope5/1  "C2"
  PS-Simulink Converter9/1 -> Scope5/2  "C1"
  PS-Simulink Converter10/1 -> Scope7/1  "F2"
  PS-Simulink Converter11/1 -> Scope7/2  "F1"
  PS-Simulink Converter12/1 -> Scope3/2  "T1"
  PS-Simulink Converter13/1 -> Scope9/1  "F1"
  Transport Delay/1 -> Scope1/1, Simulink-PS Converter/1
  connections:
  Hydraulic Reference/LConn1 -- Solver Configuration/RConn1 -- Hydraulic Fluid/RConn1 -- Hydraulic Constant Flow Rate Source/RConn1
  Hydraulic Constant Flow Rate Source/LConn1 -- Check Valve2/LConn1 -- Pressure Relief Valve/LConn1
  Pressure Relief Valve1/RConn1 -- 4-Way Directional Valve3/RConn3 -- 4-Way Directional Valve2/RConn3 -- 4-Way Directional Valve1/RConn3 -- Pressure Relief Valve/RConn1 -- "Filter "/LConn1 -- Check Valve1/LConn1
  Check Valve1/RConn1 -- Hydraulic Reference1/LConn1 -- "Filter "/RConn1
  Check Valve3/LConn1 -- Feed/RConn2 -- Hydraulic Pressure Sensor4/LConn1 -- Pressure Relief Valve3/RConn1
  Mass/LConn1 -- Translational Damper/LConn1 -- Feed/RConn1 -- Ideal Translational Motion Sensor/LConn1
  Mechanical Translational Reference/LConn1 -- Feed/LConn1
  Simulink-PS Converter/RConn1 -- 4-Way Directional Valve3/RConn1 -- 4-Way Directional Valve2/RConn1 -- 4-Way Directional Valve1/RConn1
  Translational Damper/RConn1 -- Ideal Translational Motion Sensor/RConn1 -- Mechanical Translational Reference2/LConn1
  PS-Simulink Converter2/LConn1 -- Ideal Translational Motion Sensor/RConn3
  PS-Simulink Converter1/LConn1 -- Ideal Translational Motion Sensor/RConn2
  4-Way Directional Valve2/LConn2 -- Hydraulic Pressure Sensor1/LConn1 -- Check Valve4/RConn1 -- Pressure Relief Valve2/LConn1
  Check Valve4/LConn1 -- Pressure Relief Valve2/RConn1 -- Clamp/RConn2
  Mechanical Translational Reference3/LConn1 -- Clamp/LConn1
  Mechanical Translational Reference6/LConn1 -- Cut/LConn1
  Translational Damper1/LConn1 -- Clamp/RConn1 -- Mass1/LConn1 -- Ideal Translational Motion Sensor1/LConn1
  PS-Simulink Converter7/LConn1 -- Ideal Translational Motion Sensor1/RConn3
  PS-Simulink Converter3/LConn1 -- Ideal Translational Motion Sensor1/RConn2
  Translational Damper2/LConn1 -- Cut/RConn1 -- Mass2/LConn1 -- Ideal Translational Motion Sensor2/LConn1
  Ideal Translational Motion Sensor2/RConn3 -- PS-Simulink Converter8/LConn1
  PS-Simulink Converter5/LConn1 -- Ideal Translational Motion Sensor2/RConn2
  Feed/LConn2 -- 4-Way Directional Valve1/LConn1
  Check Valve6/LConn1 -- Pressure Relief Valve5/RConn1 -- Clamp/LConn2
  4-Way Directional Valve3/LConn2 -- Cut/RConn2 -- Hydraulic Pressure Sensor/LConn1
  Check Valve5/RConn1 -- Pressure Relief Valve4/LConn1 -- 4-Way Directional Valve3/LConn1 -- Hydraulic Pressure Sensor5/LConn1
  Check Valve5/LConn1 -- Cut/LConn2 -- Pressure Relief Valve4/RConn1
  Mechanical Translational Reference1/LConn1 -- Ideal Translational Motion Sensor1/RConn1 -- Translational Damper1/RConn1
  Ideal Translational Motion Sensor2/RConn1 -- Mechanical Translational Reference4/LConn1 -- Translational Damper2/RConn1
  4-Way Directional Valve2/RConn2 -- 4-Way Directional Valve3/RConn2 -- Hydraulic Pressure Sensor6/LConn1 -- Spring-Loaded Accumulator/RConn1 -- Check Valve2/RConn1 -- Pressure Relief Valve1/LConn1 -- 4-Way Directional Valve1/RConn2
  PS-Simulink Converter4/LConn1 -- Hydraulic Pressure Sensor/RConn2
  Hydraulic Pressure Sensor/RConn1 -- Hydraulic Reference2/LConn1
  Hydraulic Pressure Sensor1/RConn1 -- Hydraulic Reference3/LConn1
  PS-Simulink Converter6/LConn1 -- Hydraulic Pressure Sensor1/RConn2
  Hydraulic Pressure Sensor2/RConn1 -- Hydraulic Reference4/LConn1
  PS-Simulink Converter9/LConn1 -- Hydraulic Pressure Sensor2/RConn2
  PS-Simulink Converter10/LConn1 -- Hydraulic Pressure Sensor3/RConn2
  Hydraulic Pressure Sensor4/RConn1 -- Hydraulic Reference6/LConn1
  PS-Simulink Converter11/LConn1 -- Hydraulic Pressure Sensor4/RConn2
  Hydraulic Pressure Sensor5/RConn1 -- Hydraulic Reference7/LConn1
  PS-Simulink Converter12/LConn1 -- Hydraulic Pressure Sensor5/RConn2
  Hydraulic Pressure Sensor3/RConn1 -- Hydraulic Reference5/LConn1
  Check Valve6/RConn1 -- 4-Way Directional Valve2/LConn1 -- Hydraulic Pressure Sensor2/LConn1 -- Pressure Relief Valve5/LConn1
  PS-Simulink Converter13/LConn1 -- Hydraulic Pressure Sensor6/RConn2
  Hydraulic Pressure Sensor6/RConn1 -- Hydraulic Reference8/LConn1
  Check Valve3/RConn1 -- Hydraulic Pressure Sensor3/LConn1 -- 4-Way Directional Valve1/LConn2 -- Pressure Relief Valve3/LConn1
